simulink model "estabilizacion_webcam"  (R2014b)
settings: Solver=ode45  StartTime=0.0  StopTime=inf  RelTol=1e-3
InitFcn:
  | webcam
values from neighbouring files (symbols this model uses):
  PosXIn = 295    [webcam.m]
  PosYIn = 225    [webcam.m]
  SearchEx = 20    [webcam.m]
  TemplateXSize = 50    [webcam.m]
  TemplateYSize = 50    [webcam.m]
undefined symbols (not defined in the file or in its folder): IsPositionTracked, IsSkeletonTracked, JointDepthIndices, JointImageIndices, JointTrackingState, JointWorldCoordinates, none, PositionDepthIndices, PositionImageIndices, PositionWorldCoordinates, SegmentationData, SkeletonTrackingID, videoinput
libraries: visionsinks x5, dspvision x2, imaqlib x1, visionutilities x1, visionanalysis x1, visiongeotforms x1
settings Model: Creator=manuel  LastModifiedBy=manuel

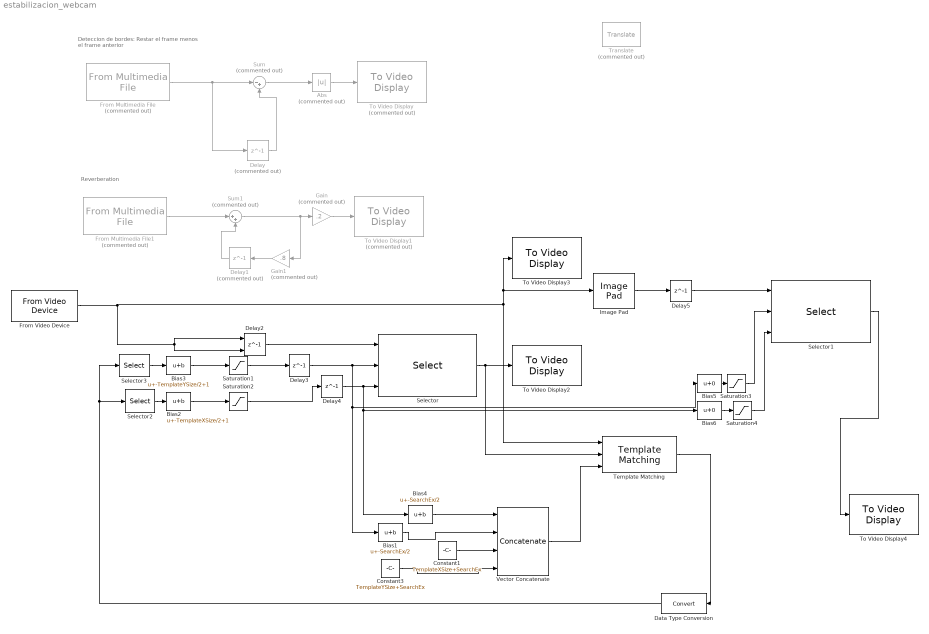
== system estabilizacion_webcam ==
  note: Deteccion de bordes:
      | Restar el frame menos el frame anterior
  note: Reverberation
  Abs : Abs  Commented=on
  Bias1 : Bias  Bias=-SearchEx/2
  Bias2 : Bias  Bias=-TemplateXSize/2+1  SaturateOnIntegerOverflow=on
  Bias3 : Bias  Bias=-TemplateYSize/2+1
  Bias4 : Bias  Bias=-SearchEx/2
  Bias5 : Bias
  Bias6 : Bias
  Constant1 : Constant  Value=TemplateXSize+SearchEx
  Constant3 : Constant  Value=TemplateYSize+SearchEx
  Data Type Conversion : DataTypeConversion
  Delay : Delay  Commented=on  DelayLength=1  InitialCondition=0
  Delay1 : Delay  Commented=on  DelayLength=1  InitialCondition=0
  Delay2 : Delay  DelayLength=1  InitialConditionSource=Input port  InitialCondition=0
      settings: InputPortMap=u0,p4
  Delay3 : Delay  DelayLength=1  InitialCondition=PosYIn
  Delay4 : Delay  DelayLength=1  InitialCondition=PosXIn
  Delay5 : Delay  DelayLength=1  InitialCondition=0
  From Multimedia File : dspvision/From Multimedia File  Commented=on  inputFilename=C:\Program Files (x86)\MATLAB\R2014b\toolbox\vision\visiondemos\shaky_car.avi  loop=on  numPlays=inf  outputStreams=Video only  videoDataType=single  audioDataType=int16  inheritSampleTime=on  userDefinedSampleTime=1/30  noAudioOutput=off  isIntensityVideo=off  fourcc=Intensity  colorVideoFormat=One multidimensional signal  outputEOF=off  dataOrg=Column-major  audioFrameSize=1024  computeAudioFrameSize=off  outSamplingMode=Sample based
  From Multimedia File1 : dspvision/From Multimedia File  Commented=on  inputFilename=C:\Program Files (x86)\MATLAB\R2014b\toolbox\vision\visiondemos\shaky_car.avi  loop=on  numPlays=inf  outputStreams=Video only  videoDataType=single  audioDataType=int16  inheritSampleTime=on  userDefinedSampleTime=1/30  noAudioOutput=off  isIntensityVideo=off  fourcc=Intensity  colorVideoFormat=One multidimensional signal  outputEOF=off  dataOrg=Column-major  audioFrameSize=1024  computeAudioFrameSize=off  outSamplingMode=Sample based
  From Video Device : imaqlib/From Video Device  DeviceMenu=winvideo 1 (Integrated Webcam)  Device=winvideo 1 (Integrated Webcam)  ObjConstructor=videoinput('winvideo', 1)  VideoFormatMenu=YUY2_640x480  VideoFormat=YUY2_640x480  VideoSource=input1  ROIPosition=[0 0 480 640]  EnableHWTrigger=off  TriggerConfiguration=none/none  SampleTime=1/30  OutputPortsMode=One multidimensional signal  DataType=single  CanDoHWTrigger=no  ReturnedColorSpace=grayscale  BlockHandle=1921.0006  ROIWidth=640  ROIHeight=480  ROIColumn=0  ROIRow=0  EngXMLPath=C:\Program Files (x86)\MATLAB\R2014b\toolbox\imaq\imaq\private  DevXMLPath=C:\MATLAB\SupportPackages\R2014b\osgenericvideointerface\toolbox\imaq\supportpackages\genericvideo\adaptor\win32  EngLibPath=C:\Program Files (x86)\MATLAB\R2014b\toolbox\imaq\imaqblks\imaqmex\win32  ColorSpace=grayscale  BayerSensorAlignment=grbg  AllMetadata=IsPositionTracked;IsSkeletonTracked;JointDepthIndices;JointImageIndices;JointTrackingState;JointWorldCoordinates;PositionDepthIndices;PositionImageIndices;PositionWorldCoordinates;SegmentationData;SkeletonTrackingID
  Gain : Gain  Commented=on  Gain=.2
  Gain1 : Gain  Commented=on  Gain=.8
  Image Pad : visionutilities/Image Pad  method=Constant  valSrc=Specify via dialog  value=0.5  spec=Pad size  rowDirection=Both left and right  outRowsMode=User-specified  rowSize=200  outColSize=10  colDirection=Both top and bottom  outColsMode=User-specified  colSize=200  outRowSize=12  trunc_flag=None
  Saturation1 : Saturate  UpperLimit=429  LowerLimit=1
  Saturation2 : Saturate  UpperLimit=589  LowerLimit=1
  Saturation3 : Saturate  UpperLimit=300  LowerLimit=1
  Saturation4 : Saturate  UpperLimit=400  LowerLimit=1
  Selector : Selector  NumberOfDimensions=2  InputPortWidth=3  IndexOptions=Starting index (port),Starting index (port)  Indices=[1 3],1  OutputSizes=TemplateYSize,TemplateXSize
  Selector1 : Selector  NumberOfDimensions=2  InputPortWidth=3  IndexOptions=Starting index (port),Starting index (port)  Indices=[1 3],1  OutputSizes=300,500
  Selector2 : Selector  InputPortWidth=2  Indices=[1]
  Selector3 : Selector  InputPortWidth=2  Indices=[2]
  Sum : Sum  Commented=on  Inputs=|-+
  Sum1 : Sum  Commented=on  Inputs=|++
  Template Matching : visionanalysis/Template Matching  metric=Sum of absolute differences  output=Best match location  method=Exhaustive  nMetric=off  nSize=3  roi=on  roiValid=off  accumMode=Binary point scaling  accumWordLength=32  accumFracLength=0  prodOutputMode=Binary point scaling  prodOutputWordLength=32  prodOutputFracLength=0  roundingMode=Floor  overflowMode=off
  To Video Display : visionsinks/To Video Display  Commented=on  inputType=Obsolete  imagePorts=One multidimensional signal  OutputDevice=On-screen video monitor  fullScreen=off  videoWindowX=467  videoWindowY=194  saveWindowSize=off  videoWindowWidth=320  videoWindowHeight=240  dataOrg=Column-major  openAtMdlStart=on  isWindowOpen=off  inputColorFormat=RGB
  To Video Display1 : visionsinks/To Video Display  Commented=on  inputType=Obsolete  imagePorts=One multidimensional signal  OutputDevice=On-screen video monitor  fullScreen=off  videoWindowX=66  videoWindowY=267  saveWindowSize=off  videoWindowWidth=320  videoWindowHeight=240  dataOrg=Column-major  openAtMdlStart=on  isWindowOpen=off  inputColorFormat=RGB
  To Video Display2 : visionsinks/To Video Display  inputType=Obsolete  imagePorts=One multidimensional signal  OutputDevice=On-screen video monitor  fullScreen=off  videoWindowX=905  videoWindowY=512  saveWindowSize=off  videoWindowWidth=120  videoWindowHeight=50  dataOrg=Column-major  openAtMdlStart=on  isWindowOpen=on  inputColorFormat=RGB
  To Video Display3 : visionsinks/To Video Display  inputType=Obsolete  imagePorts=One multidimensional signal  OutputDevice=On-screen video monitor  fullScreen=off  videoWindowX=82  videoWindowY=45  saveWindowSize=off  videoWindowWidth=640  videoWindowHeight=480  dataOrg=Column-major  openAtMdlStart=on  isWindowOpen=on  inputColorFormat=RGB
  To Video Display4 : visionsinks/To Video Display  inputType=Obsolete  imagePorts=One multidimensional signal  OutputDevice=On-screen video monitor  fullScreen=off  videoWindowX=756  videoWindowY=42  saveWindowSize=off  videoWindowWidth=500  videoWindowHeight=300  dataOrg=Column-major  openAtMdlStart=on  isWindowOpen=on  inputColorFormat=RGB
  Translate : visiongeotforms/Translate  Commented=on  outSizeT=Full  src_trans=Specify via dialog  translation="[1.5  2.3]"  maxOffset=[8 10]  fillVal=0  interpMethod=Bilinear  prodOutputMode=Binary point scaling  prodOutputWordLength=32  prodOutputFracLength=10  roundingMode=Nearest  overflowMode=on
  Vector Concatenate : Concatenate  NumInputs=4
  wires:
  Delay/1 -> Sum/2
  From Multimedia File/1 -> Delay/1, Sum/1
  Sum/1 -> Abs/1
  Abs/1 -> To Video Display/1
  From Multimedia File1/1 -> Sum1/1
  Sum1/1 -> Gain1/1, Gain/1
  Delay1/1 -> Sum1/2
  Gain/1 -> To Video Display1/1
  Gain1/1 -> Delay1/1
  Selector/1 -> Template Matching/2, To Video Display2/1
  Template Matching/1 -> Data Type Conversion/1
  From Video Device/1 -> Template Matching/1, To Video Display3/1, Image Pad/1, Delay2/2, Delay2/1
  Selector2/1 -> Bias2/1
  Selector3/1 -> Bias3/1
  Bias3/1 -> Saturation1/1
  Bias2/1 -> Saturation2/1
  Constant1/1 -> Vector Concatenate/3
  Constant3/1 -> Vector Concatenate/4
  Delay4/1 -> Bias4/1, Bias6/1, Selector/3
  Delay3/1 -> Bias5/1, Bias1/1, Selector/2
  Data Type Conversion/1 -> Selector3/1, Selector2/1
  Bias4/1 -> Vector Concatenate/1
  Bias1/1 -> Vector Concatenate/2
  Delay2/1 -> Selector/1
  Vector Concatenate/1 -> Template Matching/3
  Image Pad/1 -> Delay5/1
  Bias6/1 -> Saturation4/1
  Saturation1/1 -> Delay3/1
  Bias5/1 -> Saturation3/1
  Saturation3/1 -> Selector1/2
  Saturation4/1 -> Selector1/3
  Saturation2/1 -> Delay4/1
  Delay5/1 -> Selector1/1
  Selector1/1 -> To Video Display4/1
